simulink model "Sistema"  (R2025b)
settings: Solver=ode1  StartTime=0.0  StopTime=50  FixedStep=0.1  RelTol=1e-3  AbsTol=1e-3
settings SolverCC: AutoScaleAbsTol=off  AlgebraicLoopSolver=TrustRegion  MaxZcPerStep=1.0
settings DebuggingCC: UnconnectedInputMsg=warning  UnconnectedOutputMsg=warning  UnconnectedLineMsg=warning  SymbolicDimsDataTypeCodeGenerationDiagnostic=none
settings ModelReferenceCC: EnableRefExpFcnMdlSchedulingChecks=on
settings SFSimCC: CustomCodeUndefinedFunction=UseInterfaceOnly
settings RTWCC: GPUComputeCapability=3.5  DLArmComputeVersion=19.05
settings SimscapeCC: SimscapeLogType=all  SimscapeLogSimulationStatistics=on  SimscapeLogDataHistory=10000.0

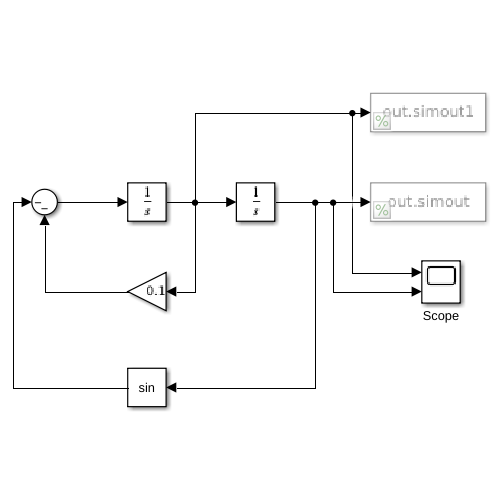
[thumbnail: Simulink's stored preview of the top-level diagram]
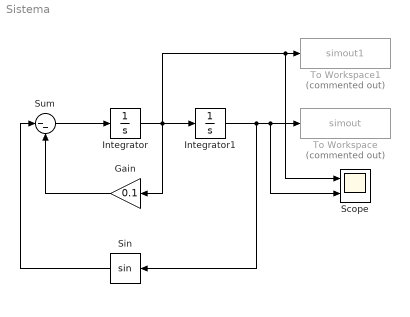
== system Sistema ==
  Gain : Gain  Gain=0.1
  Integrator : Integrator
  Integrator1 : Integrator  InitialCondition=1
  Scope : Scope  NumInputPorts=2
      settings: ActiveDisplayYMinimum=-1.6780033867316853  ActiveDisplayYMaximum=1.6645965401013969
  Sin : Trigonometry
  Sum : Sum  Inputs=|--
  To Workspace : ToWorkspace  Commented=on  VariableName=simout  SaveFormat=Timeseries  SampleTime=-1
  To Workspace1 : ToWorkspace  Commented=on  VariableName=simout1  SaveFormat=Timeseries  SampleTime=-1
  wires:
  Sum/1 -> Integrator/1
  Gain/1 -> Sum/2
  Sin/1 -> Sum/1
  Integrator/1 -> Scope/1, To Workspace1/1, Gain/1, Integrator1/1
  Integrator1/1 -> Sin/1, Scope/2, To Workspace/1
